simulink model "T_2_1"  (R2021a)
settings: Solver=VariableStepAuto  StartTime=0.0  StopTime=2  RelTol=1e-3
values from neighbouring files (symbols this model uses):
  A = [2 6; 1 0]    [t_2.m]
  B = [4; 1]    [t_2.m]
  C = [2 0]    [t_2.m]
  K = K_k*P    [t_2.m]
settings Model: Creator=fedor  LastModifiedBy=fedor

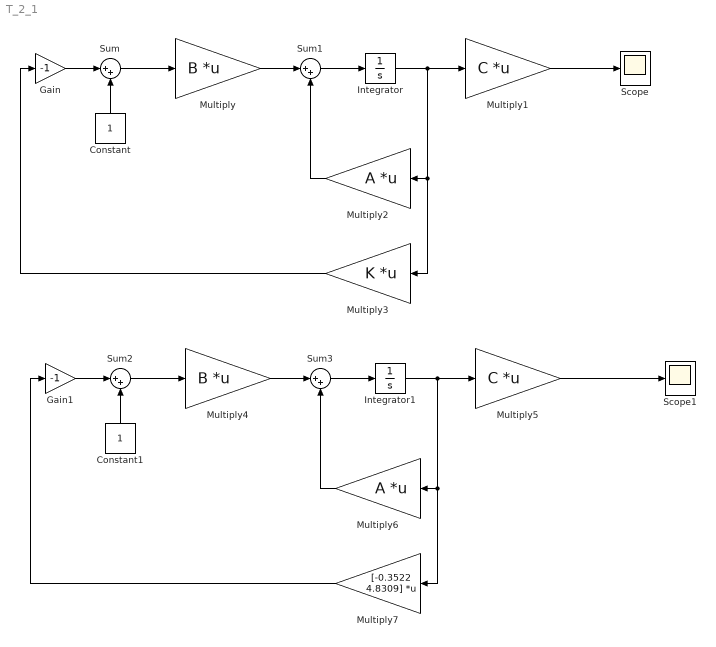
== system T_2_1 ==
  Constant : Constant
  Constant1 : Constant
  Gain : Gain  Gain=-1
  Gain1 : Gain  Gain=-1
  Integrator : Integrator
  Integrator1 : Integrator
  Multiply : Gain  Gain=B  Multiplication=Matrix(K*u)
  Multiply1 : Gain  Gain=C  Multiplication=Matrix(K*u)
  Multiply2 : Gain  Gain=A  Multiplication=Matrix(K*u)
  Multiply3 : Gain  Gain=K  Multiplication=Matrix(K*u)
  Multiply4 : Gain  Gain=B  Multiplication=Matrix(K*u)
  Multiply5 : Gain  Gain=C  Multiplication=Matrix(K*u)
  Multiply6 : Gain  Gain=A  Multiplication=Matrix(K*u)
  Multiply7 : Gain  Gain=[-0.3522 4.8309]  Multiplication=Matrix(K*u)
  Scope : Scope
  Scope1 : Scope
  Sum{,1..3} (4 alike) : Sum  Inputs=|++
  wires:
  Sum/1 -> Multiply/1
  Gain/1 -> Sum/1
  Constant/1 -> Sum/2
  Multiply/1 -> Sum1/1
  Integrator/1 -> Multiply3/1, Multiply2/1, Multiply1/1
  Sum1/1 -> Integrator/1
  Multiply2/1 -> Sum1/2
  Multiply1/1 -> Scope/1
  Multiply3/1 -> Gain/1
  Multiply7/1 -> Gain1/1
  Multiply6/1 -> Sum3/2
  Sum3/1 -> Integrator1/1
  Integrator1/1 -> Multiply5/1, Multiply6/1, Multiply7/1
  Multiply4/1 -> Sum3/1
  Constant1/1 -> Sum2/2
  Gain1/1 -> Sum2/1
  Sum2/1 -> Multiply4/1
  Multiply5/1 -> Scope1/1
